simulink model "throttle_step1"  (R2023a)
settings: Solver=VariableStepAuto  StartTime=0.0  StopTime=10.0  RelTol=1e-3
undefined symbols (not defined in the file or in its folder): degConv
settings Model: Creator=wkmiao  LastModifiedBy=wkmiao
settings DataIOCC: LoadExternalInput=on  SaveFormat=Array  ReturnWorkspaceOutputs=off

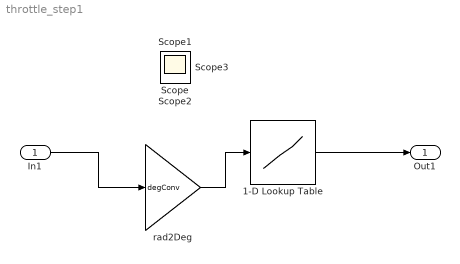
== system throttle_step1 ==
  In1 : Inport
  1-D Lookup Table : Lookup_n-D  NumberOfTableDimensions=1  BreakpointsForDimension1=[0 90]  Table=[0.5,4.5]  InternalRulePriority=Speed  RndMeth=Simplest
  rad2Deg : Gain  Gain=degConv
  Out1 : Outport
  Scope{,1..3} (4 alike) : Scope
  wires:
  In1/1 -> rad2Deg/1
  rad2Deg/1 -> 1-D Lookup Table/1
  1-D Lookup Table/1 -> Out1/1
